simulink model "sampleModel249"  (R2021b)
settings: Solver=VariableStepAuto  StartTime=0.0  StopTime=10.0  RelTol=1e-3
undefined symbols (not defined in the file or in its folder): DiscIntNeverNeededParam, Newton, Raphson
libraries: simulink x9, slpidlib x1
settings Model: Creator=user  LastModifiedBy=user

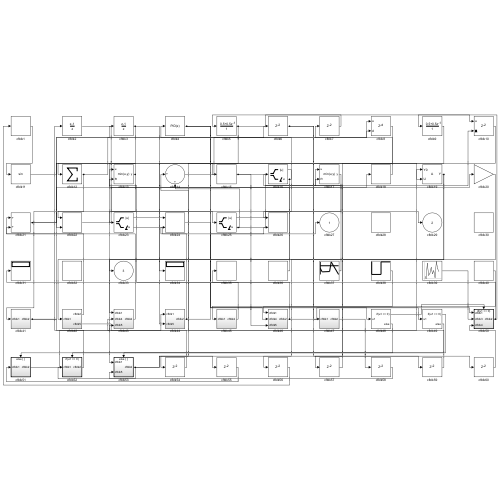
[thumbnail: Simulink's stored preview of the top-level diagram]
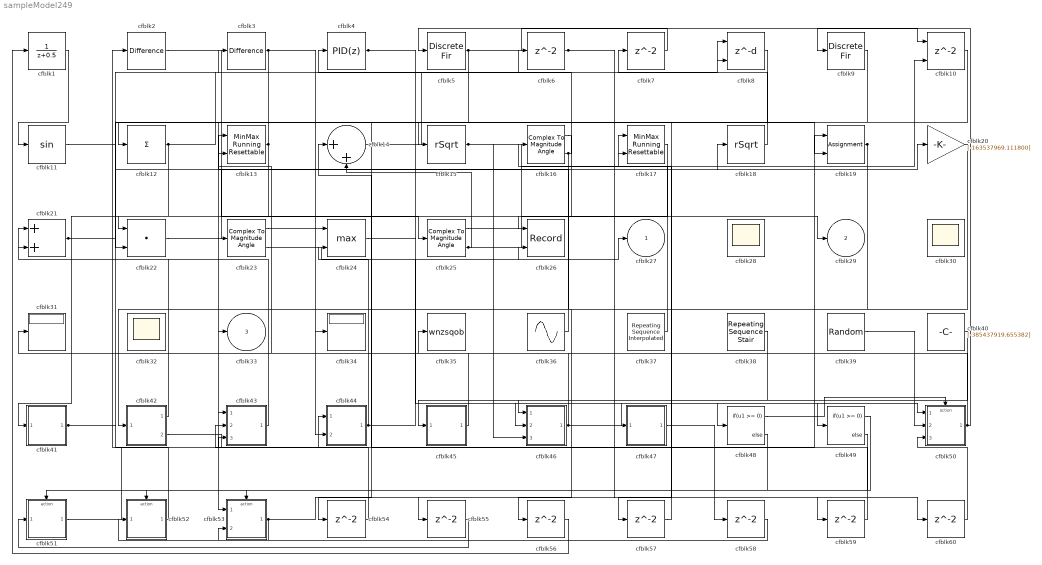
== system sampleModel249 ==
  cfblk1 : DiscreteTransferFcn  SampleTime=1
  cfblk10 : Delay  ShowEnablePort=on  SampleTime=1
      settings: InputPortMap=u0,e6
  cfblk11 : Trigonometry
  cfblk12 : Sum  Inputs=+
  cfblk13 : simulink/Math Operations/MinMax Running Resettable  Function=min  vinit=0.0
  cfblk14 : Sum  Inputs=|++
  cfblk15 : Sqrt  Operator=rSqrt  AlgorithmType=Newton-Raphson  SaturateOnIntegerOverflow=on
  cfblk16 : ComplexToMagnitudeAngle
  cfblk17 : simulink/Math Operations/MinMax Running Resettable  Function=min  vinit=0.0
  cfblk18 : Sqrt  Operator=rSqrt  AlgorithmType=Newton-Raphson  SaturateOnIntegerOverflow=on
  cfblk19 : Assignment  DiagnosticForDimensions=Warning  IndexOptions=Index vector (dialog)  Indices=1  OutputSizes=1
  cfblk2 : simulink/Discrete/Difference  ICPrevInput=0.0  OutMin=[]  OutMax=[]  OutDataTypeStr=Inherit: Inherit via back propagation  OutDataType=fixdt(1, 16)  OutScaling=2^-10  DoSatur=off
  cfblk20 : Gain  Gain=[-163537969.111800]
  cfblk21 : Sum
  cfblk22 : DotProduct  InputSameDT=on  OutDataTypeStr=Inherit: Inherit via internal rule
  cfblk23 : ComplexToMagnitudeAngle
  cfblk24 : MinMax  Function=max  Inputs=2
  cfblk25 : ComplexToMagnitudeAngle
  cfblk26 : Record  FileSettingsInternal="{\"entries\":[{\"content\":{\"excelSettings\":{\"content\":{},\"type\":\"Streamout.ExcelSettings\"}},\"type\":\"Streamout.FileSettingStorage\",\"uuid\":\"6e2f0423-9d94-49ed-921e-b4cee53c69ae\"}],\"packageUris\":[\"http://schema.mathworks.com/mf0/streamout_blocks/R2020a\"],\"version\":\"1.0\"}"  Layout=[1 1]  SignalsInternal="{\"entries\":[{\"content\":{\"signals\":[{\"content\":{\"blockPath\":[\"sampleModel249/cfblk26\"],\"channel\":[],\"dimensions\":[1],\"domain\":\"sampleModel249/cfblk26\",\"lineColor\":\"#a2142f\",\"plots\":[1],\"port\":1,\"sid\":[\"\"],\"signalID\":10075,\"signalName\":\"cfblk16:1\"},\"type\":\"RecordBlkView.Signal\",\"uuid\":\"b5ba7e04-05e0-48dd-9488-e1aff4e69d61\"},{\"content\":{\"blockPath\":[\"sampleModel249/cfblk26\"],\"channel\":[],\"dimensions\":[1],\"domain\":\"sampleModel249/cfblk26\",\"lineColor\":\"#139fff\",\"plots\":[1],\"port\":2,\"sid\":[\"\"],\"signalID\":10079,\"signalName\":\"cfblk23:2\"},\"type\":\"RecordBlkView.Signal\",\"uuid\":\"55cd0c2c-9226-4a94-837a-f9d2be7db20e\"}]},\"type\":\"RecordBlkView.InputSignals\",\"uuid\":\"9a90ef35-81a1-4567-a2b0-708c9295d5cf\"}],\"packageUris\":[\"http://schema.mathworks.com/mf0/streamout_blocks/R2020a\"],\"version\":\"1.0\"}"  VisualizationBindings="{\"xyplotplugin\":{\"info\":[{\"series\":[{\"bindingParametersList\":[{\"parameter\":\"X-Axis\",\"signalID\":10075,\"signalName\":\"cfblk16:1\"},{\"parameter\":\"Y-Axis\",\"signalID\":10079,\"signalName\":\"cfblk23:2\"}],\"seriesID\":3476}],\"subplotID\":1}]}}"  CompatibilityTag=XY
  cfblk28 : Scope
      settings: Floating=on
  cfblk3 : simulink/Discrete/Difference  ICPrevInput=0.0  OutMin=[]  OutMax=[]  OutDataTypeStr=Inherit: Inherit via back propagation  OutDataType=fixdt(1, 16)  OutScaling=2^-10  DoSatur=off
  cfblk30 : Scope
      settings: Floating=on
  cfblk31 : Display
  cfblk32 : Scope
      settings: Floating=on
  cfblk34 : Display
  cfblk35 : ToWorkspace  VariableName=wnzsqob  SaveFormat=Timeseries  SampleTime=-1
  cfblk36 : Sin  Amplitude=[-760788028.459496]  Bias=[-820139065.383940]  SampleTime=0
  cfblk37 : simulink/Sources/Repeating Sequence Interpolated  OutValues=[-261123173.442438, -618385310.378618, -587512632.754278, 398722586.552313, -873219535.010808]  TimeValues=[0 0.1 0.5 0.6 1].'  LookUpMeth=Use Input Nearest  tsamp=0.01  OutMin=[]  OutMax=[]  OutDataTypeStr=double  OutputDataTypeScalingMode=double  OutDataType=fixdt(0,8)  OutScaling=2^-10
  cfblk38 : simulink/Sources/Repeating Sequence Stair  OutValues=[-610166681.233341, -112113875.491957]  tsamp=-1  OutMin=[]  OutMax=[]  OutDataTypeStr=double  OutputDataTypeScalingMode=double  OutDataType=fixdt(0,8)  ConRadixGroup=Best Precision: Vector-wise  OutScaling=2^-12
  cfblk39 : UniformRandomNumber  Minimum=[-5478625437.297426]  Maximum=[1142133837.843585]  Seed=[39530813.000000]  SampleTime=0.1
  cfblk4 : slpidlib/PID Controller  Controller=PID  Form=Parallel  TimeDomain=Discrete-time  UseExternalTs=off  SampleTime=1  IntegratorMethod=Forward Euler  FilterMethod=Forward Euler  ControllerParametersSource=internal  P=1  I=1  D=0  UseFilter=on  N=100  TunerSelectOption=Transfer Function Based (PID Tuner App)  InitialConditionSource=internal  InitialConditionForIntegrator=0  InitialConditionForFilter=0  DifferentiatorICPrevScaledInput=0  ExternalReset=none  TrackingMode=off  Kt=1  LimitOutput=off  SatLimitsSource=internal  UpperSaturationLimit=inf  LowerSaturationLimit=-inf  LinearizeAsGain=off  AntiWindupMode=none  Kb=1  POutMin=[]  POutMax=[]  IOutMin=[]  IOutMax=[]  DOutMin=[]  DOutMax=[]  NOutMin=[]  NOutMax=[]  SumOutMin=[]  SumOutMax=[]  SaturationOutMin=[]  SaturationOutMax=[]  PParamMin=[]  PParamMax=[]  IParamMin=[]  IParamMax=[]  DParamMin=[]  DParamMax=[]  NParamMin=[]  NParamMax=[]  KbParamMin=[]  KbParamMax=[]  KtParamMin=[]  KtParamMax=[]  KbOutMin=[]  KbOutMax=[]  KtOutMin=[]  KtOutMax=[]  IntegratorOutMin=[]  IntegratorOutMax=[]  FilterOutMin=[]  FilterOutMax=[]  SumI1OutMin=[]  SumI1OutMax=[]  SumI2OutMin=[]  SumI2OutMax=[]  SumI3OutMin=[]  SumI3OutMax=[]  SumI4OutMin=[]  SumI4OutMax=[]  SumDOutMin=[]  SumDOutMax=[]  DifferentiatorOutMin=[]  DifferentiatorOutMax=[]  FilterDiffOutCoefMin=[]  FilterDiffOutCoefMax=[]  ReciprocalOutMin=[]  ReciprocalOutMax=[]  SumDenOutMin=[]  SumDenOutMax=[]  SumNumOutMin=[]  SumNumOutMax=[]  DivideOutMin=[]  DivideOutMax=[]  UdiffTsProdOutMin=[]  UdiffTsProdOutMax=[]  NTsProdOutMin=[]  NTsProdOutMax=[]  UintegralTsProdOutMin=[]  UintegralTsProdOutMax=[]  UngainTsProdOutMin=[]  UngainTsProdOutMax=[]  IntegratorContinuousStateAttributes=''  IntegratorStateMustResolveToSignalObject=off  IntegratorRTWStateStorageClass=Auto  FilterContinuousStateAttributes=''  FilterStateMustResolveToSignalObject=off  FilterRTWStateStorageClass=Auto  ParallelPVariant=InternalParameters  IdealPVariant=Disabled  IVariant=InternalParameters  DVariant=InternalParameters  IntegratorVariant=Discrete  SatVariant=Disabled  AWVariant=Passthrough  PCopyVariant=Disabled  TRVariant=Disabled  FdbkBlocksVariant=Forward  IdealPFdbkVariant=Disabled  SatFdbkVariant=Disabled  DerivativeFilterVariant=ForwardEulerFilter  NVariant=InternalParameters  NCopyVariant=Disabled  FilterICVariant=InternalICsFilter  IntegratorICVariant=InternalICs  ExternalResetVariant=Disabled  TRSumVariant=Passthrough  SumFdbkVariant=Disabled  SumVariant=Sum_PID  TsampFilterVariant=InternalTs  TsampNgainVariant=Passthrough  TsampIntegralVariant=Passthrough  ExternalSaturationOutDataTypeStr=Inherit: Same as second input
  cfblk40 : Constant  Value=[-385437919.655382]  SampleTime=1
  cfblk41 : Subsystem
  cfblk42 : Subsystem
  cfblk43 : Subsystem
  cfblk44 : Subsystem
  cfblk45 : Subsystem
  cfblk46 : Subsystem
  cfblk47 : Subsystem
  cfblk48 : If  IfExpression=u1 >= 0  SampleTime=1
  cfblk49 : If  IfExpression=u1 >= 0  SampleTime=1
  cfblk5 : DiscreteFir  SampleTime=1
  cfblk50 : Subsystem  TreatAsAtomicUnit=on
  cfblk51 : Subsystem  TreatAsAtomicUnit=on
  cfblk52 : Subsystem  TreatAsAtomicUnit=on
  cfblk53 : Subsystem  TreatAsAtomicUnit=on
  cfblk{6..7,54..60} (9 alike) : Delay  SampleTime=1
  cfblk8 : Delay  DelayLengthSource=Input port  SampleTime=1
      settings: InputPortMap=u0,p1
  cfblk9 : DiscreteFir  SampleTime=1
  cfblk27 : Outport
  cfblk29 : Outport  Port=2
  cfblk33 : Outport  Port=3
  wires:
  cfblk20/1 -> cfblk53/1(cfblk1)
  cfblk23/1 -> cfblk24/1
  cfblk1/1 -> cfblk11/1
  cfblk53/1(cfblk2) -> cfblk52/1(cfblk1), cfblk55/1, cfblk60/1
  cfblk9/1 -> cfblk43/1(cfblk1)
  cfblk46/1(cfblk2) -> cfblk49/1, cfblk13/2
  cfblk3/1 -> cfblk34/1, cfblk22/2
  cfblk38/1 -> cfblk45/1(cfblk1)
  cfblk15/1 -> cfblk17/1, cfblk46/3(cfblk5)
  cfblk50/1(cfblk2) -> cfblk9/1, cfblk35/1
  cfblk13/1 -> cfblk12/1, cfblk41/1(cfblk1)
  cfblk2/1 -> cfblk25/1
  cfblk19/1 -> cfblk33/1, cfblk56/1
  cfblk22/1 -> cfblk20/1
  cfblk52/1(cfblk2) -> cfblk2/1
  cfblk12/1 -> cfblk22/1, cfblk8/2
  cfblk18/1 -> cfblk7/1
  cfblk45/1(cfblk2) -> cfblk31/1
  cfblk36/1 -> cfblk13/1
  cfblk37/1 -> cfblk16/1
  cfblk24/1 -> cfblk50/1(cfblk1)
  cfblk39/1 -> cfblk50/2(cfblk3)
  cfblk7/1 -> cfblk5/1
  cfblk4/1 -> cfblk48/1, cfblk46/2(cfblk4), cfblk19/2
  cfblk25/1 -> cfblk29/1
  cfblk5/1 -> cfblk10/1, cfblk44/2(cfblk5)
  cfblk14/1 -> cfblk6/1
  cfblk25/2 -> cfblk10/2, cfblk14/2
  cfblk16/1 -> cfblk26/1
  cfblk11/1 -> cfblk15/1
  cfblk23/2 -> cfblk26/2
  cfblk17/1 -> cfblk23/1
  cfblk42/1(cfblk2) -> cfblk21/1
  cfblk40/1 -> cfblk46/1(cfblk1)
  cfblk43/1(cfblk2) -> cfblk21/2
  cfblk16/2 -> cfblk42/1(cfblk1), cfblk4/1
  cfblk51/1(cfblk2) -> cfblk19/1
  cfblk42/2(cfblk5) -> cfblk44/1(cfblk1)
  cfblk44/1(cfblk2) -> cfblk27/1, cfblk24/2
  cfblk21/1 -> cfblk8/1, cfblk3/1
  cfblk41/1(cfblk2) -> cfblk43/3(cfblk5), cfblk18/1
  cfblk6/1 -> cfblk47/1(cfblk1), cfblk59/1
  cfblk48/1 -> cfblk50/Action
  cfblk48/2 -> cfblk51/Action
  cfblk49/1 -> cfblk52/Action
  cfblk49/2 -> cfblk53/Action
  cfblk8/1 -> cfblk54/1
  cfblk54/1 -> cfblk43/2(cfblk4)
  cfblk55/1 -> cfblk51/1(cfblk1)
  cfblk56/1 -> cfblk1/1
  cfblk10/1 -> cfblk57/1
  cfblk57/1 -> cfblk17/2
  cfblk47/1(cfblk2) -> cfblk58/1
  cfblk58/1 -> cfblk53/2(cfblk5)
  cfblk59/1 -> cfblk14/1
  cfblk60/1 -> cfblk50/3(cfblk4)

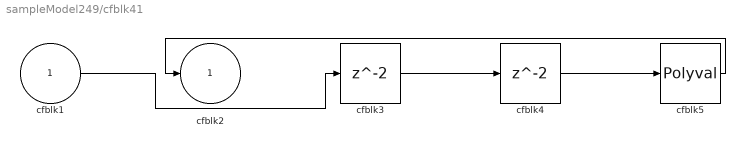
== system sampleModel249/cfblk41 ==
  cfblk1 : Inport
  cfblk3 : Delay  SampleTime=1
  cfblk4 : Delay  SampleTime=1
  cfblk5 : Polyval  Coefs=[ +2.081618890e-019, -1.441693666e-014, +4.719686976e-010, -8.536869453e-006, +1.621573104e-001, -8.087801117e+001 ]
  cfblk2 : Outport
  wires:
  cfblk5/1 -> cfblk2/1
  cfblk1/1 -> cfblk3/1
  cfblk4/1 -> cfblk5/1
  cfblk3/1 -> cfblk4/1

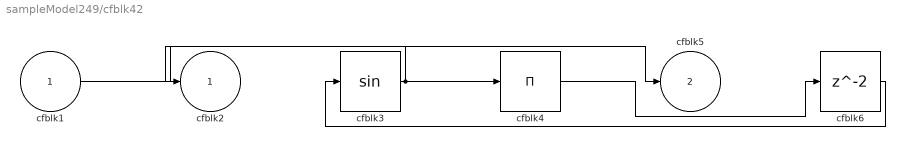
== system sampleModel249/cfblk42 ==
  cfblk1 : Inport
  cfblk3 : Trigonometry
  cfblk4 : Product  Inputs=*
  cfblk6 : Delay  SampleTime=1
  cfblk2 : Outport
  cfblk5 : Outport  Port=2
  wires:
  cfblk3/1 -> cfblk4/1, cfblk2/1
  cfblk1/1 -> cfblk5/1
  cfblk4/1 -> cfblk6/1
  cfblk6/1 -> cfblk3/1

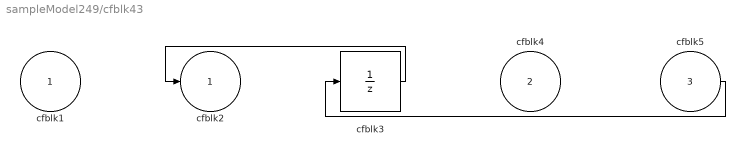
== system sampleModel249/cfblk43 ==
  cfblk1 : Inport
  cfblk4 : Inport  Port=2
  cfblk5 : Inport  Port=3
  cfblk3 : UnitDelay  HasFrameUpgradeWarning=on
  cfblk2 : Outport
  wires:
  cfblk3/1 -> cfblk2/1
  cfblk5/1 -> cfblk3/1

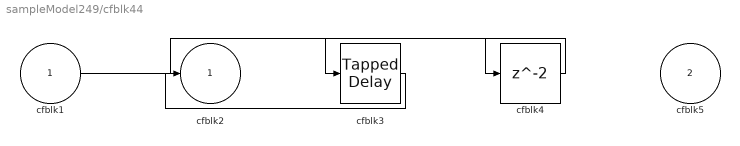
== system sampleModel249/cfblk44 ==
  cfblk1 : Inport
  cfblk5 : Inport  Port=2
  cfblk3 : simulink/Discrete/Tapped Delay  vinit=0.0  samptime=-1  NumDelays=1  DelayOrder=Oldest  includeCurrent=off
  cfblk4 : Delay  SampleTime=1
  cfblk2 : Outport
  wires:
  cfblk1/1 -> cfblk4/1
  cfblk3/1 -> cfblk2/1
  cfblk4/1 -> cfblk3/1

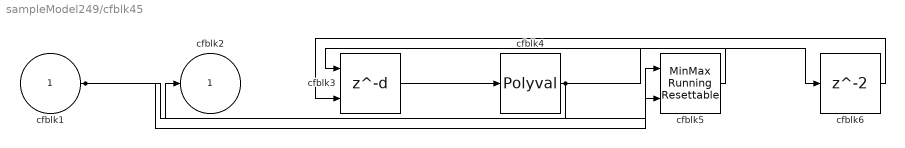
== system sampleModel249/cfblk45 ==
  cfblk1 : Inport
  cfblk3 : Delay  DelayLengthSource=Input port  SampleTime=1
      settings: InputPortMap=u0,p1
  cfblk4 : Polyval  Coefs=[ +2.081618890e-019, -1.441693666e-014, +4.719686976e-010, -8.536869453e-006, +1.621573104e-001, -8.087801117e+001 ]
  cfblk5 : simulink/Math Operations/MinMax Running Resettable  Function=min  vinit=0.0
  cfblk6 : Delay  SampleTime=1
  cfblk2 : Outport
  wires:
  cfblk5/1 -> cfblk3/1
  cfblk4/1 -> cfblk2/1, cfblk6/1
  cfblk3/1 -> cfblk4/1
  cfblk1/1 -> cfblk5/1, cfblk5/2
  cfblk6/1 -> cfblk3/2

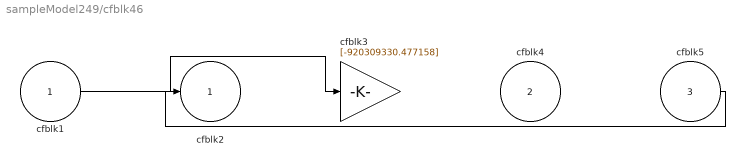
== system sampleModel249/cfblk46 ==
  cfblk1 : Inport
  cfblk4 : Inport  Port=2
  cfblk5 : Inport  Port=3
  cfblk3 : Gain  Gain=[-920309330.477158]
  cfblk2 : Outport
  wires:
  cfblk1/1 -> cfblk3/1
  cfblk5/1 -> cfblk2/1

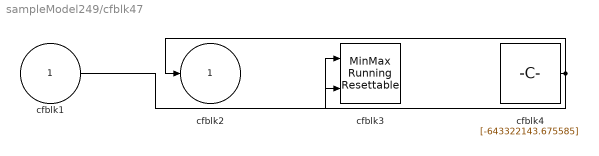
== system sampleModel249/cfblk47 ==
  cfblk1 : Inport
  cfblk3 : simulink/Math Operations/MinMax Running Resettable  Function=min  vinit=0.0
  cfblk4 : Constant  Value=[-643322143.675585]  SampleTime=1
  cfblk2 : Outport
  wires:
  cfblk4/1 -> cfblk2/1, cfblk3/2
  cfblk1/1 -> cfblk3/1

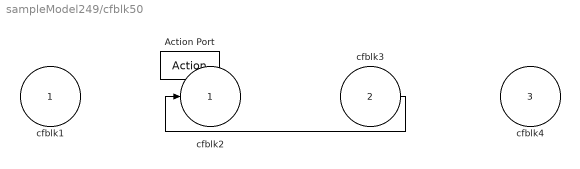
== system sampleModel249/cfblk50 ==
  cfblk1 : Inport
  cfblk3 : Inport  Port=2
  cfblk4 : Inport  Port=3
  Action Port : ActionPort  ActionPortLabel=if(u1 >= 0)
  cfblk2 : Outport
  wires:
  cfblk3/1 -> cfblk2/1

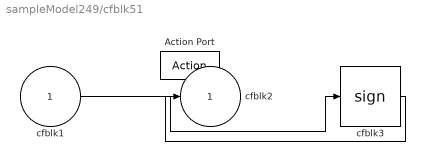
== system sampleModel249/cfblk51 ==
  cfblk1 : Inport
  Action Port : ActionPort  ActionPortLabel=else
  cfblk3 : Signum
  cfblk2 : Outport
  wires:
  cfblk1/1 -> cfblk3/1
  cfblk3/1 -> cfblk2/1

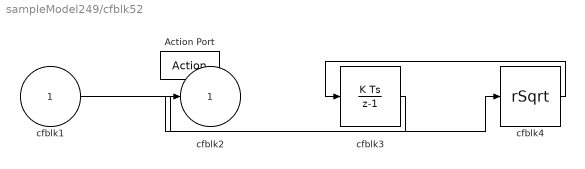
== system sampleModel249/cfblk52 ==
  cfblk1 : Inport
  Action Port : ActionPort  ActionPortLabel=if(u1 >= 0)
  cfblk3 : DiscreteIntegrator  SampleTime=-1  ICPrevOutput=DiscIntNeverNeededParam  ICPrevScaledInput=DiscIntNeverNeededParam
  cfblk4 : Sqrt  Operator=rSqrt  AlgorithmType=Newton-Raphson  SaturateOnIntegerOverflow=on
  cfblk2 : Outport
  wires:
  cfblk1/1 -> cfblk4/1
  cfblk4/1 -> cfblk3/1
  cfblk3/1 -> cfblk2/1

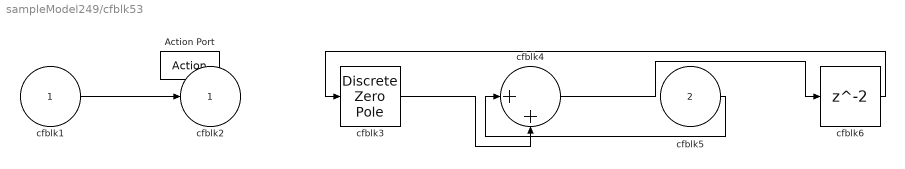
== system sampleModel249/cfblk53 ==
  cfblk1 : Inport
  cfblk5 : Inport  Port=2
  Action Port : ActionPort  ActionPortLabel=else
  cfblk3 : DiscreteZeroPole  Poles=[0 0.5]  Gain=1  SampleTime=-1
  cfblk4 : Sum  Inputs=|++
  cfblk6 : Delay
  cfblk2 : Outport
  wires:
  cfblk1/1 -> cfblk2/1
  cfblk5/1 -> cfblk4/1
  cfblk3/1 -> cfblk4/2
  cfblk4/1 -> cfblk6/1
  cfblk6/1 -> cfblk3/1
